simulink model "sop_sfun"  (R2024b)
settings: Solver=FixedStepDiscrete  StartTime=0.0  StopTime=inf  RelTol=1e-3  EnableMultiTasking=on
values from neighbouring files (symbols this model uses):
  bmsc_CellMaxVolt = 4.2    [SOP_ini.m]
  bmsc_CellMinVolt = 2.7    [SOP_ini.m]
  bmsc_InternalChgResistX = [0 23 40]    [SOP_ini.m]
  bmsc_InternalChgResistY = 0:1:100    [SOP_ini.m]
  bmsc_InternalChgResistZ = [0.026703580000000001	0.026367169999999999	0.026037069999999999	0.025713449999999999	0.025396450000000001	0.025086230000000001	0.0247829	0.024486589999999999	0.024197400000000001	0.023915410000000002	0.023640689999999999	0.0233733	0.023113290000000002	0.022860680000000001	0.022615489999999999	0.022377709999999999	0.022147340000000001	0.021924349999999999	0.021708689999999999	0.0215003	0.0212991200 ...(+1437 chars)    [SOP_ini.m]
  bmsc_InternalDischgResistX = [0 23 40]    [SOP_ini.m]
  bmsc_InternalDischgResistY = 0:1:100    [SOP_ini.m]
  bmsc_InternalDischgResistZ = [0.052496279999999999	0.050913659999999999	0.049382679999999998	0.047902229999999997	0.046471249999999999	0.045088669999999997	0.043753430000000003	0.042464509999999997	0.041220859999999998	0.04002149	0.038865379999999998	0.037751550000000002	0.036679030000000001	0.035646850000000001	0.03465406	0.033699720000000002	0.032782899999999997	0.031902680000000003	0.03105815	0.03024843	0.02947262000000000 ...(+1487 chars)    [SOP_ini.m]
  bmsc_NumberInPara = 1    [SOP_ini.m]
  bmsc_NumberInSeries = 40    [SOP_ini.m]
  sopc_ChargeDerate = 0.9    [SOP_ini.m]
  sopc_ChgFaultDerate = 0.5    [SOP_ini.m]
  sopc_DischargeDerate = 0.9    [SOP_ini.m]
  sopc_DischgFaultDerate = 0.5    [SOP_ini.m]
  sopc_SOCVsOCVX = 0:1:100    [SOP_ini.m]
  sopc_SOCVsOCVY = [2.9254229999999999 ... (first row only)    [SOP_ini.m]
settings Model: TunableVars=bmsc_CellMaxVolt,bmsc_CellMinVolt,bmsc_InternalChgResistX,bmsc_InternalChgResistY,bmsc_InternalChgResistZ,bmsc_InternalDischgResistX,bmsc_InternalDischgResistY,bmsc_InternalDischgResistZ,bmsc_NumberInPara,bmsc_NumberInSeries,sopc_ChargeDerate,sopc_ChgFaultDerate,sopc_DischargeDerate,sopc_DischgFaultDerate,sopc_SOCVsOCVX,sopc_SOCVsOCVY  TunableVarsStorageClass=Auto,Auto,Auto,Auto,Auto,Auto,Auto,Auto,Auto,Auto,Auto,Auto,Auto,Auto,Auto,Auto  TunableVarsTypeQualifier=,,,,,,,,,,,,,,,  Creator=nctzv8  LastModifiedBy=voillat
settings ConfigSet: Description=OpenECU configuration set for code generation under RTW-EC.
settings SolverCC: AlgebraicLoopSolver=TrustRegion  PositivePriorityOrder=on
settings DataIOCC: LimitDataPoints=on  SaveFormat=Array  SignalLoggingSaveFormat=ModelDataLogs
settings OptimizationCC: DefaultParameterBehavior=Inlined  InlineInvariantSignals=on  ExpressionDepthLimit=2147483647  StateBitsets=on  DataBitsets=on  ZeroExternalMemoryAtStartup=off  ZeroInternalMemoryAtStartup=off  NoFixptDivByZeroProtection=on  EfficientFloat2IntCast=on  LifeSpan=1  EfficientTunableParamExpr=on
settings DebuggingCC: SaveWithParameterizedLinksMsg=none  SignalResolutionControl=TryResolveAllWithWarning  MultiTaskDSMMsg=warning  MultiTaskCondExecSysMsg=none  SingleTaskRateTransMsg=error  CheckMatrixSingularityMsg=warning  VectorMatrixConversionMsg=warning  SignalLabelMismatchMsg=warning  UnconnectedInputMsg=warning  UnconnectedOutputMsg=warning  UnconnectedLineMsg=warning  AllowSymbolicDim=off  StateNameClashWarn=warning  SFUnexpectedBacktrackingDiag=warning  SFNoUnconditionalDefaultTransitionDiag=warning  SFExecutionAtInitializationDiag=none  ArithmeticOperatorsInVariantConditions=warning
settings HardwareCC: ProdBitPerPointer=32  ProdBitPerSizeT=32  ProdBitPerPtrDiffT=32  ProdLargestAtomicInteger=Long  ProdLargestAtomicFloat=Double  ProdEndianess=BigEndian  ProdWordSize=32  ProdHWDeviceType=Freescale->32-bit PowerPC  TargetIntDivRoundTo=Zero  TargetEndianess=BigEndian  TargetHWDeviceType=Freescale->32-bit PowerPC  ProdEqTarget=off
settings ModelReferenceCC: EnableRefExpFcnMdlSchedulingChecks=on  PropagateSignalLabelsOutOfModel=off
settings SFSimCC: SimUseLocalCustomCode=off  MATLABDynamicMemAlloc=off  CustomCodeUndefinedFunction=UseInterfaceOnly
settings RTWCC: Description=OpenECU Platform Target (ERT, optimised floating-point code)  SystemTargetFile=openecu_ert.tlc  MakeCommand=make_rtw optimized_floating_point=1  TemplateMakefile=openecu_ert_r2015b_64.tmf  RetainRTWFile=on  RTWUseLocalCustomCode=off  IncludeHyperlinkInReport=on  GPUComputeCapability=3.5
settings CodeAppCC: ForceParamTrailComments=on  IgnoreCustomStorageClasses=off  SimulinkDataObjDesc=on  CustomSymbolStrType=$N$R$M  InsertBlockDesc=on  StateflowObjectComments=on  InternalIdentifier=Classic
settings STFCustomTargetCC: TargetLibSuffix=.a  GenerateSampleERTMain=on  IncludeMdlTerminateFcn=off  CombineOutputUpdateFcns=on  IncludeFileDelimiter=UseQuote  ERTCustomFileBanners=on  SupportContinuousTime=off  RemoveResetFunc=on  MATLABClassNameForMDSCustomization=Simulink.SoftwareTarget.ERTCustomization  SystemTargetFile=openecu_ert.tlc
settings ERTTargetCC: MultiwordLength=2048  GenerateSampleERTMain=on  ParMdlRefBuildCompliant=off  CompOptLevelCompliant=off  ConcurrentExecutionCompliant=off  IncludeMdlTerminateFcn=off  IncludeFileDelimiter=UseQuote  SupportNonInlinedSFcns=on  ModelStepFunctionPrototypeControlCompliant=off  CPPClassGenCompliant=off  UseToolchainInfoCompliant=off  ExtModeMexFile=noextcomm  ERTSrcFileBannerTemplate=oe_code_c_template.cgt  ERTHdrFileBannerTemplate=oe_code_h_template.cgt  ERTDataSrcFileTemplate=oe_data_c_template.cgt  ERTDataHdrFileTemplate=oe_data_h_template.cgt  ERTCustomFileTemplate=example_file_process.tlc  GlobalDataDefinition=InSeparateSourceFile  GlobalDataReference=InSeparateHeaderFile  ConvertIfToSwitch=off  SuppressUnreachableDefaultCases=off  EnableUserReplacementTypes=on  DynamicArrayContainerType=coder::array
settings ConfigComp: CovMetricSettings=dw  CovSaveCumulativeToWorkspaceVar=on  CovSaveSingleToWorkspaceVar=on  CovExternalEMLEnable=off

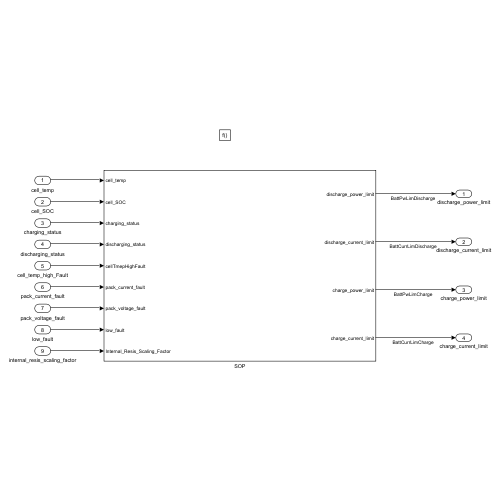
[thumbnail: Simulink's stored preview of the top-level diagram]
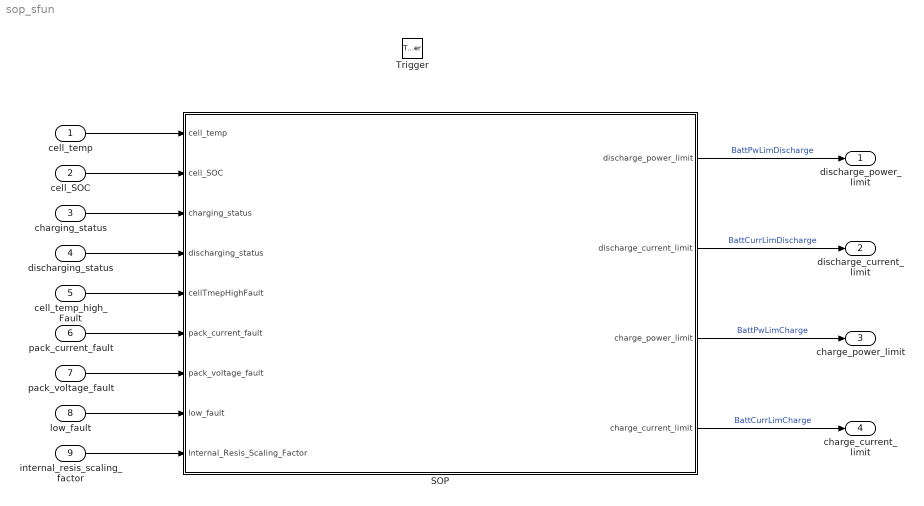
== system sop_sfun ==
  cell_temp : Inport  PortDimensions=40
  cell_SOC : Inport  Port=2  PortDimensions=40
  charging_status : Inport  Port=3
  discharging_status : Inport  Port=4
  cell_temp_high_Fault : Inport  Port=5
  pack_current_fault : Inport  Port=6
  pack_voltage_fault : Inport  Port=7
  low_fault : Inport  Port=8
  internal_resis_scaling_factor : Inport  Port=9  PortDimensions=40
  Trigger : TriggerPort  TriggerType=function-call  VariantControl=(inherit)  PortDimensions=1
  SOP : Subsystem  mask{prm_to_disp=[1..10], sfcnParam1=bmsc_CellMaxVolt, sfcnParam2=bmsc_CellMinVolt, sfcnParam3=bmsc_InternalChgResistX, sfcnParam4=bmsc_InternalChgResistY, sfcnParam5=bmsc_InternalChgResistZ, sfcnParam6=bmsc_InternalDischgResistX, sfcnParam7=bmsc_InternalDischgResistY, sfcnParam8=bmsc_InternalDischgResistZ, sfcnParam9=bmsc_NumberInPara, sfcnParam10=bmsc_NumberInSeries, sfcnParam11=sopc_ChargeDerate, sfcnParam12=sopc_ChgFaultDerate, sfcnParam13=sopc_DischargeDerate, sfcnParam14=sopc_DischgFaultDerate, sfcnParam15=sopc_SOCVsOCVX, sfcnParam16=sopc_SOCVsOCVY}
      mask prompts: prm_to_disp "Display S-function Parameters:"; sfcnParam1 "bmsc_CellMaxVolt:"; sfcnParam2 "bmsc_CellMinVolt:"; sfcnParam3 "bmsc_InternalChgResistX:"; sfcnParam4 "bmsc_InternalChgResistY:"; sfcnParam5 "bmsc_InternalChgResistZ:"; sfcnParam6 "bmsc_InternalDischgResistX:"; sfcnParam7 "bmsc_InternalDischgResistY:"; sfcnParam8 "bmsc_InternalDischgResistZ:"; sfcnParam9 "bmsc_NumberInPara:"; sfcnParam10 "bmsc_NumberInSeries:"; sfcnParam11 "sopc_ChargeDerate:"; sfcnParam12 "sopc_ChgFaultDerate:"; sfcnParam13 "sopc_DischargeDerate:"; sfcnParam14 "sopc_DischgFaultDerate:"; sfcnParam15 "sopc_SOCVsOCVX:"; sfcnParam16 "sopc_SOCVsOCVY:"
      mask help: Simulink:masks:GenSFuncDesc_MD
      mask Help: eval('feval(''rtwprivate'',''rtwhelpview'',''rtw_sfcn_block'')');
      mask TypeOptions prm_to_disp: [1..10] | [11..16]
      mask Callback prm_to_disp: slmaskprmdispcntrl(gcbh)
  discharge_power_limit : Outport
  discharge_current_limit : Outport  Port=2
  charge_power_limit : Outport  Port=3
  charge_current_limit : Outport  Port=4
  wires:
  cell_temp/1 -> SOP/1(cell_temp)
  cell_SOC/1 -> SOP/2(cell_SOC)
  charging_status/1 -> SOP/3(charging_status)
  discharging_status/1 -> SOP/4(discharging_status)
  cell_temp_high_Fault/1 -> SOP/5(cellTmepHighFault)
  pack_current_fault/1 -> SOP/6(pack_current_fault)
  pack_voltage_fault/1 -> SOP/7(pack_voltage_fault)
  internal_resis_scaling_factor/1 -> SOP/9(Internal_Resis_Scaling_Factor)
  low_fault/1 -> SOP/8(low_fault)
  SOP/1(discharge_power_limit) -> discharge_power_limit/1  "BattPwLimDischarge"
  SOP/2(discharge_current_limit) -> discharge_current_limit/1  "BattCurrLimDischarge"
  SOP/3(charge_power_limit) -> charge_power_limit/1  "BattPwLimCharge"
  SOP/4(charge_current_limit) -> charge_current_limit/1  "BattCurrLimCharge"

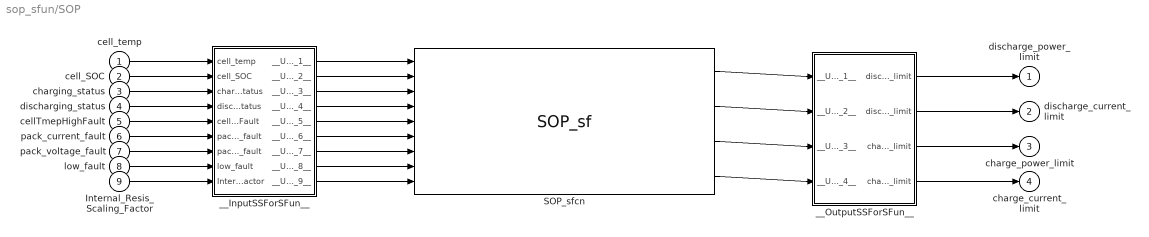
== system sop_sfun/SOP ==
  cell_temp : Inport
  cell_SOC : Inport  Port=2
  charging_status : Inport  Port=3
  discharging_status : Inport  Port=4
  cellTmepHighFault : Inport  Port=5  OutDataTypeStr=uint8
  pack_current_fault : Inport  Port=6  OutDataTypeStr=uint8
  pack_voltage_fault : Inport  Port=7  OutDataTypeStr=uint8
  low_fault : Inport  Port=8  OutDataTypeStr=uint8
  Internal_Resis_Scaling_Factor : Inport  Port=9
  SOP_sfcn : S-Function  FunctionName=SOP_sf  Parameters=sfcnParam1, sfcnParam2, sfcnParam3, sfcnParam4, sfcnParam5, sfcnParam6, sfcnParam7, sfcnParam8, sfcnParam9, sfcnParam10, sfcnParam11, sfcnParam12, sfcnParam13, sfcnParam14, sfcnParam15, sfcnParam16  SFunctionModules=""  SFunctionDeploymentMode=off  EnableBusSupport=off  mask{rtw_sf_name=SOP_sf, showVar=off, prm_to_disp=[1..10], sfcnParam1=sfcnParam1, sfcnParam2=sfcnParam2, sfcnParam3=sfcnParam3, sfcnParam4=sfcnParam4, sfcnParam5=sfcnParam5, sfcnParam6=sfcnParam6, sfcnParam7=sfcnParam7, sfcnParam8=sfcnParam8, sfcnParam9=sfcnParam9, sfcnParam10=sfcnParam10, sfcnParam11=sfcnParam11, sfcnParam12=sfcnParam12, sfcnParam13=sfcnParam13, sfcnParam14=sfcnParam14, sfcnParam15=sfcnParam15, sfcnParam16=sfcnParam16}
      mask prompts: rtw_sf_name "Simulink:masks:GenSFuncName_MP"; showVar "Simulink:masks:GenSFuncShowModuleList_MP"; prm_to_disp "Display S-function Parameters:"; sfcnParam1 "bmsc_CellMaxVolt:"; sfcnParam2 "bmsc_CellMinVolt:"; sfcnParam3 "bmsc_InternalChgResistX:"; sfcnParam4 "bmsc_InternalChgResistY:"; sfcnParam5 "bmsc_InternalChgResistZ:"; sfcnParam6 "bmsc_InternalDischgResistX:"; sfcnParam7 "bmsc_InternalDischgResistY:"; sfcnParam8 "bmsc_InternalDischgResistZ:"; sfcnParam9 "bmsc_NumberInPara:"; sfcnParam10 "bmsc_NumberInSeries:"; sfcnParam11 "sopc_ChargeDerate:"; sfcnParam12 "sopc_ChgFaultDerate:"; sfcnParam13 "sopc_DischargeDerate:"; sfcnParam14 "sopc_DischgFaultDerate:"; sfcnParam15 "sopc_SOCVsOCVX:"; sfcnParam16 "sopc_SOCVsOCVY:"
      mask help: Simulink:masks:GenSFuncDesc_MD
      mask init:
      | displist = '';
      | if ~strcmp(get_param(gcb, 'FunctionName'), rtw_sf_name);
      |   set_param(gcb, 'FunctionName', rtw_sf_name);
      | end
      | % Check if we are generating code
      | rtw_mode = false;
      | if strcmpi(get_param(bdroot(gcb),'SimulationStatus'),'Initializing')
      | 	rtw_mode = strcmpi(get_param(bdroot(gcb),'BuildingRTWCode'),'on') && ...
      | 		~strcmpi(get_param(bdroot(gcb),'TargetStyle'),'SimulationTarget');
      | end
      | if showVar || rtw_mode
      | 	if exist('rtwsfunc') == 2 | exist('rtwsfunc') == 6
      | 		tmplist = rtwsfunc(rtw_sf_name,gcb);
      | 		tmplist = DAStudio.message('Simulink:masks:GenSFuncListOfModules_IC', tmplist);
      | 	elseif showVar
      | 		tmplist1 = DAStudio.message('Simulink:masks:GenSFuncListOfModules_IC', '');
      |         tmplist2 = DAStudio.message('Simulink:masks:GenSFuncNotLicensed_IC');
      |         tmplist = [tmplist1 tmplist2];
      |  	end
      | end
      | if showVar
      |   displist = tmplist;
      | end
      settings: CopyFcn=|
      | if ~strcmp(get_param(gcb,'Linkstatus'),'none') && ...
      | ~strcmp(get_param(gcb,'Linkstatus'),'implicit')
      |   set_param(gcb,'LinkStatus','none');
      | end
      mask Help: eval('feval(''rtwprivate'',''rtwhelpview'',''rtw_sfcn_block'')');
      mask TypeOptions prm_to_disp: [1..10] | [11..16]
      mask Callback prm_to_disp: slmaskprmdispcntrl(gcbh)
      mask Display:
      | port_label('input',1,'cell_temp');
      | port_label('input',2,'cell_SOC');
      | port_label('input',3,'charging_status');
      | port_label('input',4,'discharging_status');
      | port_label('input',5,'cellTmepHighFault');
      | port_label('input',6,'pack_current_fault');
      | port_label('input',7,'pack_voltage_fault');
      | port_label('input',8,'low_fault');
      | port_label('input',9,'Internal_Resis_Scaling_Factor');
      | port_label('output',1,'discharge_power_limit');
      | port_label('output',2,'discharge_current_limit');
      | port_label('output',3,'charge_power_limit');
      | port_label('output',4,'charge_current_limit');
  __InputSSForSFun__ : Subsystem
  __OutputSSForSFun__ : Subsystem
  discharge_power_limit : Outport
  discharge_current_limit : Outport  Port=2
  charge_power_limit : Outport  Port=3
  charge_current_limit : Outport  Port=4
  wires:
  cell_temp/1 -> __InputSSForSFun__/1(cell_temp)
  cell_SOC/1 -> __InputSSForSFun__/2(cell_SOC)
  charging_status/1 -> __InputSSForSFun__/3(charging_status)
  discharging_status/1 -> __InputSSForSFun__/4(discharging_status)
  cellTmepHighFault/1 -> __InputSSForSFun__/5(cellTmepHighFault)
  pack_current_fault/1 -> __InputSSForSFun__/6(pack_current_fault)
  pack_voltage_fault/1 -> __InputSSForSFun__/7(pack_voltage_fault)
  low_fault/1 -> __InputSSForSFun__/8(low_fault)
  Internal_Resis_Scaling_Factor/1 -> __InputSSForSFun__/9(Internal_Resis_Scaling_Factor)
  __InputSSForSFun__/1(__UniqueOutportName__1__) -> SOP_sfcn/1
  __InputSSForSFun__/2(__UniqueOutportName__2__) -> SOP_sfcn/2
  __InputSSForSFun__/3(__UniqueOutportName__3__) -> SOP_sfcn/3
  __InputSSForSFun__/4(__UniqueOutportName__4__) -> SOP_sfcn/4
  __InputSSForSFun__/5(__UniqueOutportName__5__) -> SOP_sfcn/5
  __InputSSForSFun__/6(__UniqueOutportName__6__) -> SOP_sfcn/6
  __InputSSForSFun__/7(__UniqueOutportName__7__) -> SOP_sfcn/7
  __InputSSForSFun__/8(__UniqueOutportName__8__) -> SOP_sfcn/8
  __InputSSForSFun__/9(__UniqueOutportName__9__) -> SOP_sfcn/9
  SOP_sfcn/1 -> __OutputSSForSFun__/1(__UniqueInportName__1__)
  SOP_sfcn/2 -> __OutputSSForSFun__/2(__UniqueInportName__2__)
  SOP_sfcn/3 -> __OutputSSForSFun__/3(__UniqueInportName__3__)
  SOP_sfcn/4 -> __OutputSSForSFun__/4(__UniqueInportName__4__)
  __OutputSSForSFun__/1(discharge_power_limit) -> discharge_power_limit/1
  __OutputSSForSFun__/2(discharge_current_limit) -> discharge_current_limit/1
  __OutputSSForSFun__/3(charge_power_limit) -> charge_power_limit/1
  __OutputSSForSFun__/4(charge_current_limit) -> charge_current_limit/1

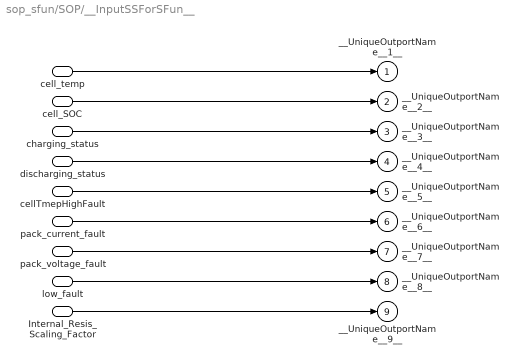
== system sop_sfun/SOP/__InputSSForSFun__ ==
  cell_temp : Inport
  cell_SOC : Inport  Port=2
  charging_status : Inport  Port=3
  discharging_status : Inport  Port=4
  cellTmepHighFault : Inport  Port=5  OutDataTypeStr=uint8
  pack_current_fault : Inport  Port=6  OutDataTypeStr=uint8
  pack_voltage_fault : Inport  Port=7  OutDataTypeStr=uint8
  low_fault : Inport  Port=8  OutDataTypeStr=uint8
  Internal_Resis_Scaling_Factor : Inport  Port=9
  __UniqueOutportName__1__ : Outport
  __UniqueOutportName__2__ : Outport  Port=2
  __UniqueOutportName__3__ : Outport  Port=3
  __UniqueOutportName__4__ : Outport  Port=4
  __UniqueOutportName__5__ : Outport  Port=5
  __UniqueOutportName__6__ : Outport  Port=6
  __UniqueOutportName__7__ : Outport  Port=7
  __UniqueOutportName__8__ : Outport  Port=8
  __UniqueOutportName__9__ : Outport  Port=9
  wires:
  cell_temp/1 -> __UniqueOutportName__1__/1
  cell_SOC/1 -> __UniqueOutportName__2__/1
  charging_status/1 -> __UniqueOutportName__3__/1
  discharging_status/1 -> __UniqueOutportName__4__/1
  cellTmepHighFault/1 -> __UniqueOutportName__5__/1
  pack_current_fault/1 -> __UniqueOutportName__6__/1
  pack_voltage_fault/1 -> __UniqueOutportName__7__/1
  low_fault/1 -> __UniqueOutportName__8__/1
  Internal_Resis_Scaling_Factor/1 -> __UniqueOutportName__9__/1

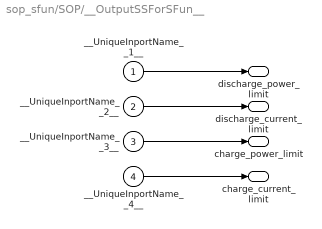
== system sop_sfun/SOP/__OutputSSForSFun__ ==
  __UniqueInportName__1__ : Inport
  __UniqueInportName__2__ : Inport  Port=2
  __UniqueInportName__3__ : Inport  Port=3
  __UniqueInportName__4__ : Inport  Port=4
  discharge_power_limit : Outport
  discharge_current_limit : Outport  Port=2
  charge_power_limit : Outport  Port=3
  charge_current_limit : Outport  Port=4
  wires:
  __UniqueInportName__1__/1 -> discharge_power_limit/1
  __UniqueInportName__2__/1 -> discharge_current_limit/1
  __UniqueInportName__3__/1 -> charge_power_limit/1
  __UniqueInportName__4__/1 -> charge_current_limit/1
